simulink model "CC"  (R2023a)
settings: Solver=VariableStepAuto  StartTime=0.0  StopTime=15  RelTol=1e-3
undefined symbols (not defined in the file): Ion, Lithium
libraries: spsBatteryLib x1, spsControlledCurrentSourceLib x1, spsMosfetLib x1, sps_lib x1
settings Model: Creator=Siddesh  LastModifiedBy=Siddesh

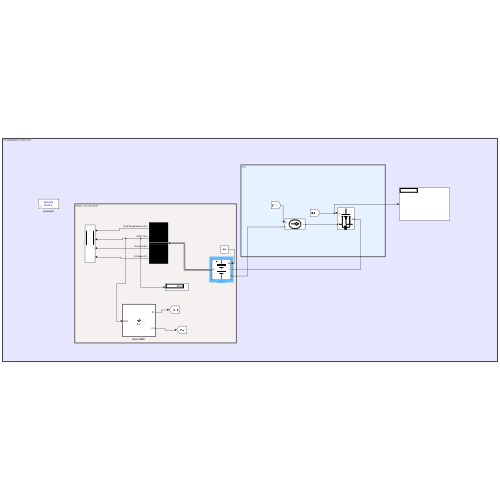
[thumbnail: Simulink's stored preview of the top-level diagram]
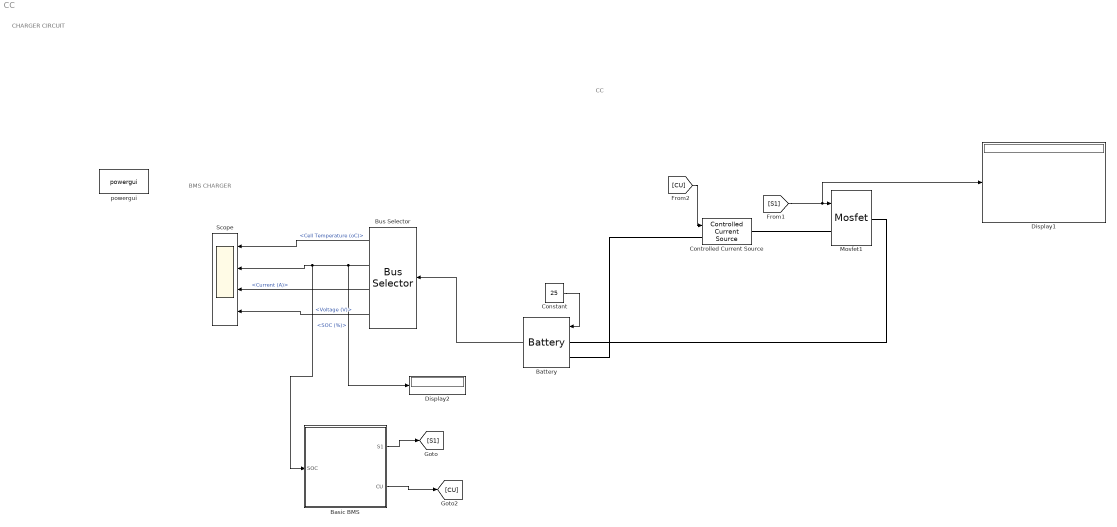
== system CC ==
  note: BMS CHARGER
  note: CC
  note: CHARGER CIRCUIT
  "Basic BMS " : MATLAB Function  TreatAsAtomicUnit=on
  Battery : spsBatteryLib/Battery  BatType=Lithium-Ion  ShowTempParam=on  ThermalPreset="3.3V  2.3Ah  (LiFePO4)"  ShowAgeParam=off  NomV=3.3  NomQ=2.3  SOC=89.99  Batt_Tr=30  PresetModel=off  MaxQ=2.3  MinV=2.475  FullV=3.748  Dis_rate=2.3  R=0.014  Normal_OP=2.25  expZone="[3.4788       0.113]"  current=[6.5 13 32.5]  Units=Time  Tci=20  NomT=25  T2=0  MaxQ2=2.208  FullV2=3.45  Normal_OP2=2.85  expZone2="[3.22       0.015]"  Rca=0.6  ti=1000  Dp=0  Neq0=0  Tsim=1e6  Ta1=25  Qeol=5.4*0.9  Reol=0.013333*1.2  Char_age=[2.3478, 3]  Dis_age=[2.3478, 10]  N1=1500  N2=10500  N3=1000  N4=1400  Ta2=45  N5=950
  Bus Selector : BusSelector  OutputSignals=Cell Temperature (oC),SOC (%),Current (A),Voltage (V)
  Constant : Constant  Value=25
  Controlled Current Source : spsControlledCurrentSourceLib/Controlled Current Source  Initialize=on  Source_Type=AC  Amplitude=0  Phase=0  Frequency=0  Measurements=None
  Display1 : Display
  Display2 : Display
  Mosfet1 : spsMosfetLib/Mosfet  Ron=0.1  Lon=0  Rd=0.01  Vfd=0  IC=0  Rs=1e5  Cs=inf  Measurements=off
  Scope : Scope  NumInputPorts=4
  powergui : sps_lib/powergui  Priority=1  SimulationMode=Discrete  SampleTime=50e-6  frequency=60  Iterations=50  frequencyindice=0  Pbase=100e6  ErrMax=1e-4  UnitsV=kV  UnitsW=MW  buscounter=0  FunctionMessages=off  echomessages=off  EnableUseOfTLC=off  CurrentSourceSwitches=off  DisableSnubberDevices=off  DisableRonSwitches=off  DisableVfSwitches=off  DisplayEquations=off  AutomaticDiscreteSolvers=off  SolverType=Tustin/Backward Euler (TBE)  Interpol=off  ExternalGateDelay=off  methode=off  Ts=100  x0status=blocks  SPID=on  SwTol=0  HookPort=off  NonlinearTolerance=1e-4  nMaxIteration=100  ContinueOnMaxIteration=off  RestoreLinks=warning  ResistiveCurrentMeasurement=off  Frange=[0:2:500]  Ylog=off  Xlog=on  ShowGrid=off  save=off  variable=ZData  structure=0  ZoomFFT=off  StartTime=0.0  cycles=1  DisplayStyle=1  fundamental=60  FreqAxis=off  MaxFrequency=1000  frequencyindicesteady=1  RmsSteady=1  display=off
  wires:
  [CU] -> Controlled Current Source/1
  "Basic BMS "/1(S1) -> [S1]
  Bus Selector/1 -> Scope/1  "<Cell Temperature (oC)>"
  Constant/1 -> Battery/1
  Bus Selector/4 -> Scope/4  "<Voltage (V)>"
  Battery/1 -> Bus Selector/1
  Bus Selector/2 -> Display2/1, "Basic BMS "/1(SOC), Scope/2  "<SOC (%)>"
  Bus Selector/3 -> Scope/3  "<Current (A)>"
  [S1] -> Display1/1, Mosfet1/1
  "Basic BMS "/2(CU) -> [CU]
  connections:
  Controlled Current Source/LConn1 -- Battery/LConn2
  Controlled Current Source/RConn1 -- Mosfet1/LConn1
  Mosfet1/RConn1 -- Battery/LConn1

== matlab function CC/Basic BMS  ==
  data: SOC input; S1 output; CU output
function [S1, CU] = fcn(SOC)

CU = 0;
if ((SOC == 0) || (SOC <= 80))
    S1 = 1;
    CU = 2;
    disp("SOC80");
elseif ((SOC >80) && (SOC <90))
    S1 = 1;
else 
    S1 = 0;
end
